simulink model "flightsim62022_withUDPJoystick"  (R2024a)
settings: Solver=ode45  StartTime=0.0  StopTime=300  FixedStep=0.02  RelTol=1e-3
undefined symbols (not defined in the file): Earth, f, WGS84
libraries: instrumentlib x3, simulink_extras x2, aerolibfltsims x2, shared6dof x1, aerolibtransform2 x1, sim3dlib x1
settings Model: Creator=naman  LastModifiedBy=Gman
settings DataIOCC: OutputSaveName=out

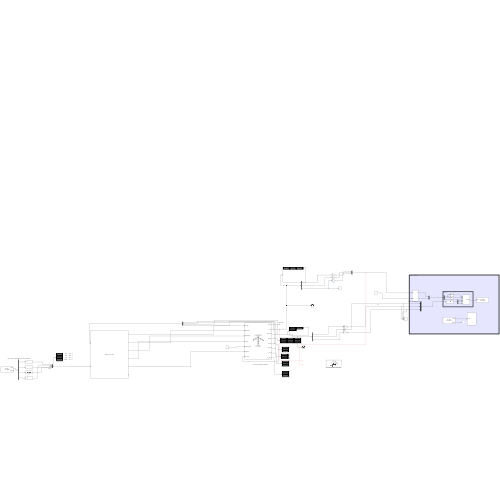
[thumbnail: Simulink's stored preview of the top-level diagram]
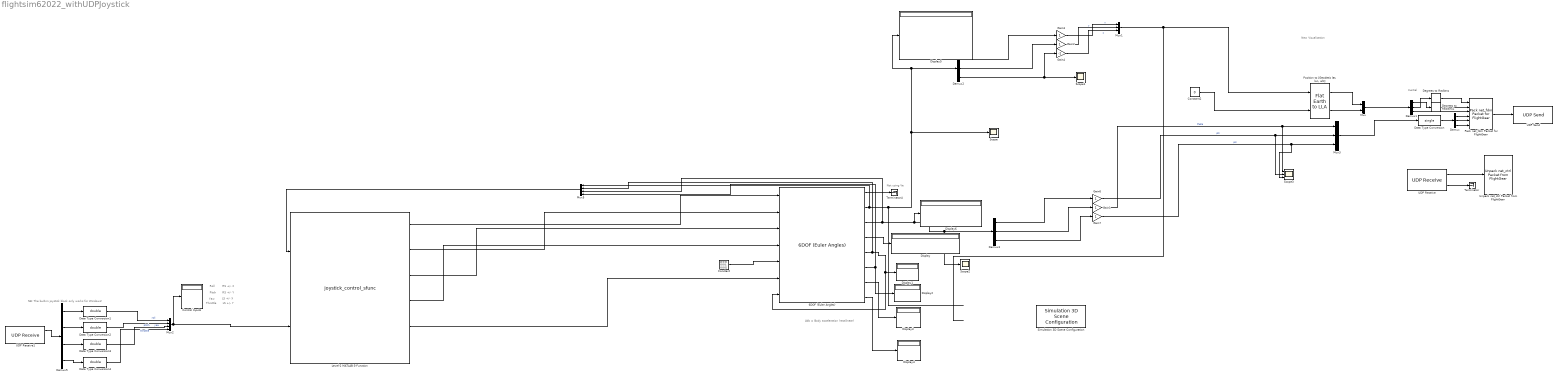
== system flightsim62022_withUDPJoystick ==
  note: NB: The built-in joystick block only works for Windows!
  note: Abb = Body acceleration (rectilinear)
  note: Not using Ve
  note: Throttle
  note: Yaw
  note: Pitch
  note: Roll
  note: LS +/- X
  note: RS +/- X
  note: RS +/- Y
  note: LS +/- Y
  note: New Visualization
  note: Inertial
  6DOF (Euler Angles) : shared6dof/6DOF (Euler Angles)  units=Metric (MKS)  mtype=Custom Variable  rep=Euler Angles  xme_0=Initialpos  Vm_0=InitialVel  eul_0=InitialOri  pm_0=InitialRot  mass_0=mass  mass_e=0.5  mass_f=2.0  inertia=Inertia  inertia_e=eye(3)  inertia_f=2*eye(3)  k_quat=1.0  vre_flag=on  abi_flag=off  aMode=0  xme_statename=''  Vm_statename=''  eul_statename=''  quat_statename=''  pm_statename=''  mass_statename=''
  Constant : Constant  Value=[0 0 0; 0 0 0; 0 0 0]
  Constant2 : Constant  Value=0
  Control Inputs : Display
  Data Type Conversion : DataTypeConversion  OutDataTypeStr=single  SaturateOnIntegerOverflow=off  RndMeth=Floor
  Data Type Conversion{1..4} (4 alike) : DataTypeConversion  OutDataTypeStr=double  SaturateOnIntegerOverflow=off  RndMeth=Floor
  Degrees to Radians : simulink_extras/Transformations/Degrees to Radians
  Degrees to Radians1 : simulink_extras/Transformations/Degrees to Radians
  Demux{,1..3} (4 alike) : Demux  Outputs=3
  Demux5 : Demux
  Display{,1..6} (7 alike) : Display
  Gain{1..3,6..7} (5 alike) : Gain
  Gain4 : Gain  Gain=-1
  Level-2 MATLAB S-Function : M-S-Function  FunctionName=joystick_control_sfunc
  Mux : Mux  Inputs=2
  Mux1 : Mux  Inputs=3
  Mux2 : Mux
  Mux3 : Mux  Inputs=3
  Mux5 : Mux
  Pack net_fdm Packet for FlightGear : aerolibfltsims/Pack net_fdm Packet for FlightGear  FlightGearVersion=v2019.1  ShowPositionAttitudeInputs=on  ShowVelocityAccelerationInputs=off  ShowControlSurfacePositionInputs=off  ShowEngineFuelInputs=off  ShowLandingGearInputs=off  ShowEnvironmentInputs=off  SampleTime=-1  packetVersion=24
  "Position to [Geodetic lat, lon, alti]" : aerolibtransform2/Flat Earth to LLA  units=Metric (MKS)  ptype=Earth (WGS84)  F=1/298.257223563  R=6378137  refPosPort=off  LL0=[37.210265015306916, -80.41446644179189]  psi=0
  Scope : Scope
  Scope1 : Scope
  Scope2 : Scope
  Scope3 : Scope  NumInputPorts=3
  Simulation 3D Scene Configuration : sim3dlib/Simulation 3D Scene Configuration  Priority=0  ProjectFormat=Default Scenes  SceneDesc=Airport  ProjectName=C:\Program Files\MATLAB\R2024a\toolbox\shared\sim3d_projects\automotive_project_windows\UE\WindowsNoEditor\VehicleSimulation.exe  ScenePath=/Game/Maps/HwStrght  EnableOpenDRIVE=off  vehTagList={'Custom';'Scene Origin';'SimulinkVehicle1'}  vehTag=SimulinkVehicle1  FreeCameraInitialTranslation=[-6, 0, 2]  FreeCameraDefaultInitialTranslation=[-6, 0, 2]  FreeCameraInitialRotation=[0, -15, 0]  FreeCameraDefaultInitialRotation=[0, -15, 0]  OpVisEn=off  Ts=1/60  EnableWindow=on  EnableRemoteAccess=off  EnableWeather=off  SunAzimuth=90  SunAltitude=40.0  EnableGeospatialSun=off  Latitude=0  Longitude=0  Date=2023-01-01  Time=10:30:00  GeoTimeZone=-5.0  SunDaylightSaving=off  wind=1  clouds=10  EnableVolumetricClouds=off  CloudCoverage=0  CloudAltitude=6  fog=0  rain=0  RaindropsEffect=off  SnowDensity=0  EnableGeospatial=off  UseTrueOrigin=off  OriginHeight=200  OriginLatitude=40.744652  OriginLongitude=-73.988864  MapStyle=Aerial  AdditionalAssetIDs=[]  UseAdvancedSunSky=off  SolarTime=11  TimeZone=-5  Day=21  Month=9  Year=2022  UseDaylightSavingTime=on  DSTStartDay=10  DSTStartMonth=3  DSTEndDay=3  DSTEndMonth=11  DSTSwitchHour=2  sensorTag=MainCamera1  sensorId=1  sensorName=MainCamera1  mountLoc=Origin  offsetFlag=off  tmountOffset=[0, 0, 0]  rmountOffset=[0, 0, 0]  HorizontalResolution=1280  VerticalResolution=720  HorizontalFOV=60  mountPoint=[0 0 0]  mountOrientation=[0 0 0]  aMode=0  ID=1  GeoTrigger=Inactive
      settings: LibrarySourceBlock=aerolibsim3d/Simulation 3D Scene Configuration
  Terminator : Terminator
  Terminator4 : Terminator
  UDP Receive : instrumentlib/UDP Receive  LocalAddress=127.0.0.1  LocalPort=50001  EnablePortSharing=off  Host=localhost  Port=65343  GetLatestData=on  DataSize=[ 1, 744 ]  DataType=uint8  ASCIIFormatting=%f,  Terminator=LF  CustomTerminator=10  ByteOrder=little-endian  EnableBlockingMode=off  Timeout=10  SampleTime=0.2  SimulateUsing=Interpreted execution
  UDP Receive1 : instrumentlib/UDP Receive  LocalAddress=127.0.0.1  LocalPort=5505  EnablePortSharing=off  Host=localhost  Port=9090  GetLatestData=on  DataSize=[ 1, 4]  DataType=single  ASCIIFormatting=%f,  Terminator=LF  CustomTerminator=10  ByteOrder=big-endian  EnableBlockingMode=off  Timeout=10  SampleTime=1/60  SimulateUsing=Interpreted execution
  UDP Send : instrumentlib/UDP Send  Host=localhost  Port=50000  LocalAddress=127.0.0.1  LocalPort=-1  EnablePortSharing=on  OutputDatagramPacketSize=4096  ByteOrder=big-endian  EnableBlockingMode=on  SimulateUsing=Interpreted execution
  Unpack net_ctrl Packet from FlightGear : aerolibfltsims/Unpack net_ctrl Packet from FlightGear  FlightGearVersion=v2019.1  ShowControlSurfacePositionOutputs=off  ShowEngineFuelOutputs=off  ShowLandingGearOutputs=off  ShowAvionicOutputs=off  ShowEnvironmentOutputs=off  SampleTime=-1  packetVersion=27
  wires:
  UDP Receive/1 -> Unpack net_ctrl Packet from FlightGear/1
  "Position to [Geodetic lat, lon, alti]"/2 -> Mux/2
  Demux/3 -> Pack net_fdm Packet for FlightGear/6
  Gain1/1 -> Scope3/1, Mux3/1  "theta"
  Demux1/2 -> Degrees to Radians/1
  Degrees to Radians1/1 -> Pack net_fdm Packet for FlightGear/2
  Gain6/1 -> Mux3/2, Scope3/2  "phi"
  Data Type Conversion/1 -> Demux/1
  Demux/1 -> Pack net_fdm Packet for FlightGear/4
  Demux/2 -> Pack net_fdm Packet for FlightGear/5
  UDP Receive/2 -> Terminator/1
  "Position to [Geodetic lat, lon, alti]"/1 -> Mux/1
  Demux1/3 -> Pack net_fdm Packet for FlightGear/3
  Gain7/1 -> Scope3/3, Mux3/3  "psi"
  Mux3/1 -> Data Type Conversion/1
  Pack net_fdm Packet for FlightGear/1 -> UDP Send/1
  Degrees to Radians/1 -> Pack net_fdm Packet for FlightGear/1
  Demux1/1 -> Degrees to Radians1/1
  Mux/1 -> Demux1/1
  6DOF (Euler Angles)/4 -> Display/1
  6DOF (Euler Angles)/3 -> Mux5/3, Display6/1, Scope2/1, Demux3/1
  Demux3/1 -> Gain6/1
  Demux3/2 -> Gain1/1
  Demux3/3 -> Gain7/1
  6DOF (Euler Angles)/5 -> Mux5/2, 6DOF (Euler Angles)/7, Display1/1
  6DOF (Euler Angles)/6 -> Mux5/4, Display2/1
  6DOF (Euler Angles)/7 -> Display3/1
  6DOF (Euler Angles)/8 -> Display4/1
  Demux2/1 -> Gain3/1
  Demux2/3 -> Scope1/1, Gain4/1
  Demux2/2 -> Gain2/1
  Gain4/1 -> Mux1/3  "z"
  Gain3/1 -> Mux1/1  "x"
  Gain2/1 -> Mux1/2  "y"
  Mux1/1 -> "Position to [Geodetic lat, lon, alti]"/1
  Constant2/1 -> "Position to [Geodetic lat, lon, alti]"/2
  6DOF (Euler Angles)/1 -> Terminator4/1
  6DOF (Euler Angles)/2 -> Mux5/1, Scope/1, Demux2/1, Display5/1
  Mux5/1 -> Level-2 MATLAB S-Function/1
  Constant/1 -> 6DOF (Euler Angles)/5
  Level-2 MATLAB S-Function/1 -> 6DOF (Euler Angles)/1
  Level-2 MATLAB S-Function/2 -> 6DOF (Euler Angles)/2
  Level-2 MATLAB S-Function/3 -> 6DOF (Euler Angles)/3
  Level-2 MATLAB S-Function/4 -> 6DOF (Euler Angles)/4
  Level-2 MATLAB S-Function/5 -> 6DOF (Euler Angles)/6
  Mux2/1 -> Control Inputs/1, Level-2 MATLAB S-Function/2
  Data Type Conversion1/1 -> Mux2/1  "roll"
  Data Type Conversion2/1 -> Mux2/2  "pitch"
  Data Type Conversion3/1 -> Mux2/3  "yaw"
  Data Type Conversion4/1 -> Mux2/4  "throttle"
  UDP Receive1/1 -> Demux5/1
  Demux5/1 -> Data Type Conversion1/1
  Demux5/2 -> Data Type Conversion2/1
  Demux5/3 -> Data Type Conversion3/1
  Demux5/4 -> Data Type Conversion4/1
